simulink model "Even_Odd"  (R2021a)
settings: Solver=FixedStepDiscrete  StartTime=0.0  StopTime=10.0  RelTol=1e-3  EnableMultiTasking=on
libraries: simulink x1
settings Model: Creator=Osman  LastModifiedBy=Osman
settings DataIOCC: ReturnWorkspaceOutputs=off
settings OptimizationCC: DefaultParameterBehavior=Inlined  InlineInvariantSignals=on  EnableMemcpy=off  LifeSpan=1  EfficientTunableParamExpr=on
settings DebuggingCC: UnderspecifiedInitializationDetection=Classic  MergeDetectMultiDrivingBlocksExec=none  SFMachineParentedDataDiag=warning  ArithmeticOperatorsInVariantConditions=warning
settings ModelReferenceCC: PropagateSignalLabelsOutOfModel=off
settings SFSimCC: MATLABDynamicMemAlloc=off  CustomCodeUndefinedFunction=UseInterfaceOnly
settings RTWCC: SystemTargetFile=ert.tlc  GenCodeOnly=on  TemplateMakefile=ert_default_tmf  GenerateReport=on  IncludeHyperlinkInReport=on  LaunchReport=on  GenerateTraceInfo=on  GenerateTraceReport=on  GenerateTraceReportSl=on  GenerateTraceReportSf=on  GenerateTraceReportEml=on
settings CodeAppCC: ForceParamTrailComments=on  IgnoreCustomStorageClasses=off  OperatorAnnotations=on  SimulinkDataObjDesc=on  SFDataObjDesc=on  MATLABFcnDesc=on  InsertBlockDesc=on  StateflowObjectComments=on  MATLABSourceComments=on
settings ERTTargetCC: MultiwordLength=2048  GenerateSampleERTMain=on  InlinedParameterPlacement=NonHierarchical  ERTCustomFileTemplate=example_file_process.tlc

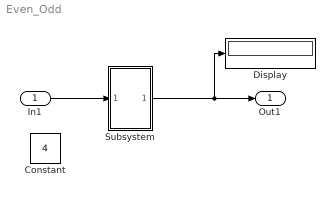
== system Even_Odd ==
  In1 : Inport  OutDataTypeStr=uint8
  Constant : Constant  Value=4  OutDataTypeStr=uint8
  Display : Display
  Subsystem : Subsystem
  Out1 : Outport
  wires:
  Subsystem/1(Out1) -> Display/1, Out1/1
  In1/1 -> Subsystem/1(In1)

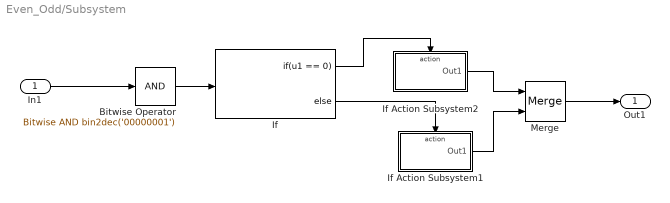
== system Even_Odd/Subsystem ==
  In1 : Inport
  Bitwise Operator : simulink/Logic and Bit Operations/Bitwise Operator  logicop=AND  UseBitMask=on  BitMask=bin2dec('00000001')  BitMaskRealWorld=Stored Integer
  If : If  IfExpression=u1 == 0
  If Action Subsystem1 : Subsystem  TreatAsAtomicUnit=on
  If Action Subsystem2 : Subsystem  TreatAsAtomicUnit=on
  Merge : Merge
  Out1 : Outport
  wires:
  If/2 -> If Action Subsystem1/Action
  If Action Subsystem2/1(Out1) -> Merge/1
  In1/1 -> Bitwise Operator/1
  Merge/1 -> Out1/1
  Bitwise Operator/1 -> If/1
  If/1 -> If Action Subsystem2/Action
  If Action Subsystem1/1(Out1) -> Merge/2

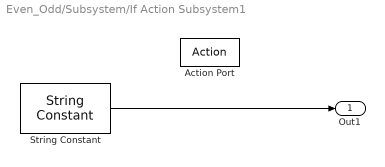
== system Even_Odd/Subsystem/If Action Subsystem1 ==
  Action Port : ActionPort  ActionPortLabel=else
  String Constant : StringConstant  String="\"Odd\""
  Out1 : Outport
  wires:
  String Constant/1 -> Out1/1

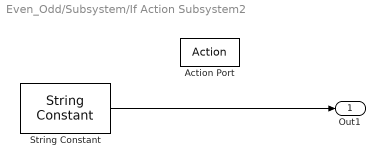
== system Even_Odd/Subsystem/If Action Subsystem2 ==
  Action Port : ActionPort  ActionPortLabel=if(u1 == 0)
  String Constant : StringConstant  String="\"Even\""
  Out1 : Outport
  wires:
  String Constant/1 -> Out1/1
